simulink model "walk2"  (R2020a)
settings: Solver=FixedStepDiscrete  StartTime=0.0  StopTime=20  FixedStep=deltaT  RelTol=1e-3
InitFcn:
  | %****NOTE: you must change the line below
  | % to the IP address for YOUR ROS master!****
  | deltaT = 0.1;
  | %ipaddress = 'http://10.4.155.40:11311'; % Tech Hall
  | ipaddress = 'http://192.168.43.20:11311'; % phone
  | 
  | % --- Start MATLAB Global Node
  | try % try to print list of ROS nodes
  |     rosnode list
  |     clc
  | % if error from rosnode list,
  | % initialize ROS global node from MATLAB
  | catch exp
  |     rosinit(ipaddress)  % only if error: rosinit
  |     pause(5)
  | end
StartFcn:
  | % Publishers to ROS topics for left, right
  | % upper arm joint commands
  | Larm = rospublisher('/darwin/j_high_arm_l_position_controller/command','std_msgs/Float64');
  | Rarm = rospublisher('/darwin/j_high_arm_r_position_controller/command','std_msgs/Float64');
  | 
  | % Create ROS messages to publishers
  | Ldown = rosmessage(Larm);
  | Rdown = rosmessage(Rarm);
  | Ldown2 = rosmessage(Larm);
  | Rdown2 = rosmessage(Rarm);
  | 
  | % move upper arm joint to 0.5 radian
  | Ldown.Data = 0.5;
  | Rdown.Data = 0.5;
  | 
  | % move upper arm joint to 0.8 radian
  | Ldown2.Data = 0.8;
  | Rdown2.Data = 0.8;
  | 
  | % move arms to 0.5 radian during two-second period,
  | % then to 0.8 radian during another
  | % two-second period (arms move synchronously)
  | send(Larm,Ldown);
  | send(Rarm,Rdown);
  | pause(2)
  | send(Larm,Ldown2);
  | send(Rarm,Rdown2);
  | pause(2)
  | 
  | disturb = rossvcclient('/gazebo/apply_body_wrench');
  | disturbmsg = rosmessage(disturb);
  | disturbmsg.ReferenceFrame = 'world';
  | disturbmsg.ReferencePoint.X = 0; disturbmsg.ReferencePoint.Y = 0; disturbmsg.ReferencePoint.Z = 0;
  | disturbmsg.Wrench.Force.X = 0.0; disturbmsg.Wrench.Force.Y = 0.0; disturbmsg.Wrench.Force.Z = 0.0;
  | disturbmsg.Wrench.Torque.X = 0.0; disturbmsg.Wrench.Torque.Y = 0.0; disturbmsg.Wrench.Torque.Z = 0.0;
  | disturbmsg.StartTime.Sec = 0; disturbmsg.StartTime.Nsec = 0;
  | disturbmsg.Duration.Sec = 0; disturbmsg.Duration.Nsec = 500000000;
StopFcn:
  | rosshutdown
model workspace (MAT data in the model file):
  SL_ROS_VariableLengthArrays_MaxSizes.CommonInfo.ArrayTruncateAction = 'EmitWarning'
  SL_ROS_VariableLengthArrays_MaxSizes.MsgTypeMap = containers.Map
  SL_ROS_VariableLengthArrays_MaxSizes.MsgTypeMap.serialization.keys = {'gazebo_msgs/ApplyBodyWrenchRequest', 'sensor_msgs/JointState'}
  SL_ROS_VariableLengthArrays_MaxSizes.MsgTypeMap.serialization.values{1}(1).PropertyName = 'BodyName'
  SL_ROS_VariableLengthArrays_MaxSizes.MsgTypeMap.serialization.values{1}(1).DataType = 'uint8'
  SL_ROS_VariableLengthArrays_MaxSizes.MsgTypeMap.serialization.values{1}(1).MaxLength = 19
  SL_ROS_VariableLengthArrays_MaxSizes.MsgTypeMap.serialization.values{1}(2).PropertyName = 'ReferenceFrame'
  SL_ROS_VariableLengthArrays_MaxSizes.MsgTypeMap.serialization.values{1}(2).DataType = 'uint8'
  SL_ROS_VariableLengthArrays_MaxSizes.MsgTypeMap.serialization.values{1}(2).MaxLength = 5
  SL_ROS_VariableLengthArrays_MaxSizes.MsgTypeMap.serialization.values{2}(1).PropertyName = 'Effort'
  SL_ROS_VariableLengthArrays_MaxSizes.MsgTypeMap.serialization.values{2}(1).DataType = 'double'
  SL_ROS_VariableLengthArrays_MaxSizes.MsgTypeMap.serialization.values{2}(1).MaxLength = 128
  SL_ROS_VariableLengthArrays_MaxSizes.MsgTypeMap.serialization.values{2}(2).PropertyName = 'Name'
  SL_ROS_VariableLengthArrays_MaxSizes.MsgTypeMap.serialization.values{2}(2).DataType = 'std_msgs/String'
  SL_ROS_VariableLengthArrays_MaxSizes.MsgTypeMap.serialization.values{2}(2).MaxLength = 24
  SL_ROS_VariableLengthArrays_MaxSizes.MsgTypeMap.serialization.values{2}(3).PropertyName = 'Position'
  SL_ROS_VariableLengthArrays_MaxSizes.MsgTypeMap.serialization.values{2}(3).DataType = 'double'
  SL_ROS_VariableLengthArrays_MaxSizes.MsgTypeMap.serialization.values{2}(3).MaxLength = 128
  SL_ROS_VariableLengthArrays_MaxSizes.MsgTypeMap.serialization.values{2}(4).PropertyName = 'Velocity'
  SL_ROS_VariableLengthArrays_MaxSizes.MsgTypeMap.serialization.values{2}(4).DataType = 'double'
  SL_ROS_VariableLengthArrays_MaxSizes.MsgTypeMap.serialization.values{2}(4).MaxLength = 128
  SL_ROS_VariableLengthArrays_MaxSizes.MsgTypeMap.serialization.uniformity = 0
  SL_ROS_VariableLengthArrays_MaxSizes.MsgTypeMap.serialization.keyType = 'char'
  SL_ROS_VariableLengthArrays_MaxSizes.MsgTypeMap.serialization.valueType = 'any'
libraries: robotlib x22, realtime_pacer_lib x1
settings Model: Creator=JerryLee  LastModifiedBy=JerryLee
settings OptimizationCC: EnhancedBackFolding=on  PassReuseOutputArgsAs=Individual arguments  ZeroExternalMemoryAtStartup=off  ZeroInternalMemoryAtStartup=off  MaxStackSize=64  OptimizeBlockOrder=speed  DifferentSizesBufferReuse=on  OptimizationCustomize=off  EfficientTunableParamExpr=on
settings DebuggingCC: ParameterTunabilityLossMsg=error
settings HardwareCC: ProdBitPerPointer=32  ProdBitPerSizeT=32  ProdBitPerPtrDiffT=32  ProdLargestAtomicFloat=None  ProdIntDivRoundTo=Undefined  ProdEndianess=Unspecified  ProdWordSize=32  ProdHWDeviceType=Generic->Unspecified (assume 32-bit Generic)  UseEmbeddedCoderFeatures=off
settings SFSimCC: MATLABDynamicMemAlloc=off
settings RTWCC: SystemTargetFile=ert.tlc  HardwareBoard=Robot Operating System (ROS)  TemplateMakefile=ert_default_tmf  Toolchain=Catkin  TargetLang=C++
settings CodeAppCC: ForceParamTrailComments=on  IgnoreCustomStorageClasses=off  OperatorAnnotations=on  SimulinkDataObjDesc=on  SFDataObjDesc=on  InsertBlockDesc=on
settings ERTTargetCC: SupportNonInlinedSFcns=on

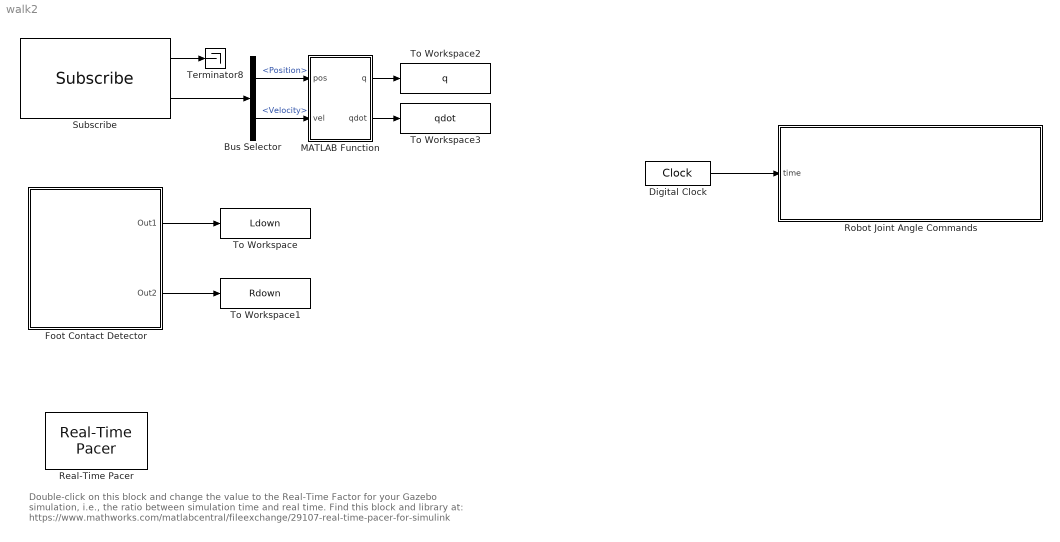
== system walk2 ==
  note: Double-click on this block and
      | change the value to the Real-Time
      | Factor for your Gazebo simulation,
      | i.e., the ratio between simulation time
      | and real time.
      |
      | Find this block and library at:
      | https://www.mathworks.com/matlabcentral/fileexchange/29107-real-time-pacer-for-simulink
  Bus Selector : BusSelector  OutputSignals=Position,Velocity
  Digital Clock : DigitalClock  SampleTime=deltaT
  Foot Contact Detector : Subsystem
  MATLAB Function : MATLAB Function  TreatAsAtomicUnit=on
  Real-Time Pacer : realtime_pacer_lib/Real-Time Pacer  simTimePerRealTime=0.5
      settings: SourceProductName=Real-Time Pacer
  Robot Joint Angle Commands : Subsystem
  Subscribe : robotlib/Subscribe  topicSource=Select from ROS network  topic=/darwin/joint_states  messageType=sensor_msgs/JointState  sampleTime=deltaT  messageQueueLength=1
  Terminator8 : Terminator
  To Workspace : ToWorkspace  VariableName=Ldown  SampleTime=deltaT
  To Workspace1 : ToWorkspace  VariableName=Rdown  SampleTime=deltaT
  To Workspace2 : ToWorkspace  VariableName=q  SampleTime=deltaT
  To Workspace3 : ToWorkspace  VariableName=qdot  SampleTime=deltaT
  wires:
  Subscribe/1 -> Terminator8/1
  Foot Contact Detector/2(Out2) -> To Workspace1/1
  Foot Contact Detector/1(Out1) -> To Workspace/1
  Subscribe/2 -> Bus Selector/1
  Digital Clock/1 -> Robot Joint Angle Commands/1(time)
  Bus Selector/1 -> MATLAB Function/1(pos)  "<Position>"
  Bus Selector/2 -> MATLAB Function/2(vel)  "<Velocity>"
  MATLAB Function/1(q) -> To Workspace2/1
  MATLAB Function/2(qdot) -> To Workspace3/1

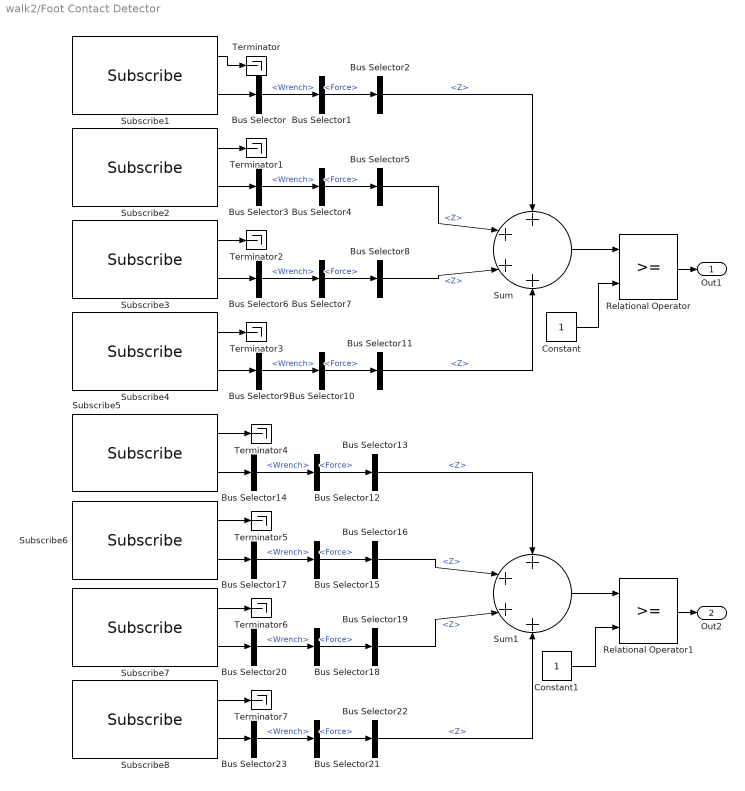
== system walk2/Foot Contact Detector ==
  Bus Selector{,3,6,9,14,17,20,23} (8 alike) : BusSelector  OutputSignals=Wrench
  Bus Selector{1,4,7,10,12,15,18,21} (8 alike) : BusSelector  OutputSignals=Force
  Bus Selector{2,5,8,11,13,16,19,22} (8 alike) : BusSelector  OutputSignals=Z
  Constant : Constant
  Constant1 : Constant
  Relational Operator : RelationalOperator  OutDataTypeStr=boolean  RndMeth=Simplest
  Relational Operator1 : RelationalOperator  OutDataTypeStr=boolean  RndMeth=Simplest
  Subscribe1 : robotlib/Subscribe  topicSource=Select from ROS network  topic=/leap_one/left_foot_sensor_m0  messageType=geometry_msgs/WrenchStamped  sampleTime=deltaT  messageQueueLength=1
  Subscribe2 : robotlib/Subscribe  topicSource=Select from ROS network  topic=/leap_one/left_foot_sensor_m1  messageType=geometry_msgs/WrenchStamped  sampleTime=deltaT  messageQueueLength=1
  Subscribe3 : robotlib/Subscribe  topicSource=Select from ROS network  topic=/leap_one/left_foot_sensor_m2  messageType=geometry_msgs/WrenchStamped  sampleTime=deltaT  messageQueueLength=1
  Subscribe4 : robotlib/Subscribe  topicSource=Select from ROS network  topic=/leap_one/left_foot_sensor_m3  messageType=geometry_msgs/WrenchStamped  sampleTime=deltaT  messageQueueLength=1
  Subscribe5 : robotlib/Subscribe  topicSource=Select from ROS network  topic=/leap_one/right_foot_sensor_m0  messageType=geometry_msgs/WrenchStamped  sampleTime=deltaT  messageQueueLength=1
  Subscribe6 : robotlib/Subscribe  topicSource=Select from ROS network  topic=/leap_one/right_foot_sensor_m1  messageType=geometry_msgs/WrenchStamped  sampleTime=deltaT  messageQueueLength=1
  Subscribe7 : robotlib/Subscribe  topicSource=Select from ROS network  topic=/leap_one/right_foot_sensor_m2  messageType=geometry_msgs/WrenchStamped  sampleTime=deltaT  messageQueueLength=1
  Subscribe8 : robotlib/Subscribe  topicSource=Select from ROS network  topic=/leap_one/right_foot_sensor_m3  messageType=geometry_msgs/WrenchStamped  sampleTime=deltaT  messageQueueLength=1
  Sum : Sum  Inputs=4
  Sum1 : Sum  Inputs=4
  Terminator{,1..7} (8 alike) : Terminator
  Out1 : Outport
  Out2 : Outport  Port=2
  wires:
  Bus Selector6/1 -> Bus Selector7/1  "<Wrench>"
  Subscribe8/2 -> Bus Selector23/1
  Bus Selector22/1 -> Sum1/4  "<Z>"
  Bus Selector8/1 -> Sum/3  "<Z>"
  Subscribe5/1 -> Terminator4/1
  Bus Selector/1 -> Bus Selector1/1  "<Wrench>"
  Subscribe1/2 -> Bus Selector/1
  Bus Selector2/1 -> Sum/1  "<Z>"
  Bus Selector20/1 -> Bus Selector18/1  "<Wrench>"
  Bus Selector19/1 -> Sum1/3  "<Z>"
  Subscribe2/2 -> Bus Selector3/1
  Bus Selector17/1 -> Bus Selector15/1  "<Wrench>"
  Constant/1 -> Relational Operator/2
  Bus Selector3/1 -> Bus Selector4/1  "<Wrench>"
  Relational Operator1/1 -> Out2/1
  Bus Selector18/1 -> Bus Selector19/1  "<Force>"
  Bus Selector9/1 -> Bus Selector10/1  "<Wrench>"
  Subscribe2/1 -> Terminator1/1
  Bus Selector4/1 -> Bus Selector5/1  "<Force>"
  Bus Selector16/1 -> Sum1/2  "<Z>"
  Subscribe7/1 -> Terminator6/1
  Relational Operator/1 -> Out1/1
  Bus Selector13/1 -> Sum1/1  "<Z>"
  Constant1/1 -> Relational Operator1/2
  Subscribe7/2 -> Bus Selector20/1
  Bus Selector23/1 -> Bus Selector21/1  "<Wrench>"
  Subscribe6/2 -> Bus Selector17/1
  Subscribe6/1 -> Terminator5/1
  Bus Selector10/1 -> Bus Selector11/1  "<Force>"
  Bus Selector21/1 -> Bus Selector22/1  "<Force>"
  Sum/1 -> Relational Operator/1
  Subscribe3/1 -> Terminator2/1
  Bus Selector11/1 -> Sum/4  "<Z>"
  Bus Selector5/1 -> Sum/2  "<Z>"
  Subscribe4/2 -> Bus Selector9/1
  Subscribe5/2 -> Bus Selector14/1
  Subscribe3/2 -> Bus Selector6/1
  Bus Selector7/1 -> Bus Selector8/1  "<Force>"
  Subscribe1/1 -> Terminator/1
  Sum1/1 -> Relational Operator1/1
  Bus Selector15/1 -> Bus Selector16/1  "<Force>"
  Bus Selector1/1 -> Bus Selector2/1  "<Force>"
  Subscribe4/1 -> Terminator3/1
  Bus Selector14/1 -> Bus Selector12/1  "<Wrench>"
  Subscribe8/1 -> Terminator7/1
  Bus Selector12/1 -> Bus Selector13/1  "<Force>"

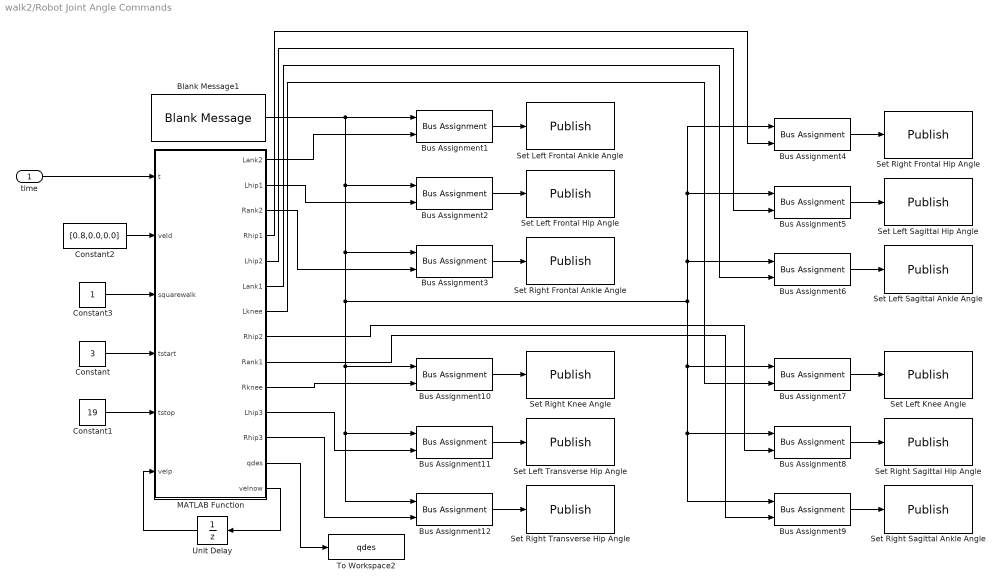
== system walk2/Robot Joint Angle Commands ==
  time : Inport
  Blank Message1 : robotlib/Blank Message  messageClass=Message  entityType=std_msgs/Float64  messageType=std_msgs/Float64  SampleTime=deltaT
  Bus Assignment{1..12} (12 alike) : BusAssignment  AssignedSignals=Data
  Constant : Constant  Value=3
  Constant1 : Constant  Value=19
  Constant2 : Constant  Value=[0.8,0.0,0.0]
  Constant3 : Constant
  MATLAB Function : MATLAB Function  TreatAsAtomicUnit=on
  Set Left Frontal Ankle Angle : robotlib/Publish  topicSource=Select from ROS network  topic=/darwin/j_ankle2_l_position_controller/command  messageType=std_msgs/Float64  messageQueueLength=1
  Set Left Frontal Hip Angle : robotlib/Publish  topicSource=Select from ROS network  topic=/darwin/j_thigh1_l_position_controller/command  messageType=std_msgs/Float64  messageQueueLength=1
  Set Left Knee Angle : robotlib/Publish  topicSource=Select from ROS network  topic=/darwin/j_tibia_l_position_controller/command  messageType=std_msgs/Float64  messageQueueLength=1
  Set Left Sagittal Ankle Angle : robotlib/Publish  topicSource=Select from ROS network  topic=/darwin/j_ankle1_l_position_controller/command  messageType=std_msgs/Float64  messageQueueLength=1
  Set Left Sagittal Hip Angle : robotlib/Publish  topicSource=Select from ROS network  topic=/darwin/j_thigh2_l_position_controller/command  messageType=std_msgs/Float64  messageQueueLength=1
  Set Left Transverse Hip Angle : robotlib/Publish  topicSource=Select from ROS network  topic=/darwin/j_pelvis_l_position_controller/command  messageType=std_msgs/Float64  messageQueueLength=1
  Set Right Frontal Ankle Angle : robotlib/Publish  topicSource=Select from ROS network  topic=/darwin/j_ankle2_r_position_controller/command  messageType=std_msgs/Float64  messageQueueLength=1
  Set Right Frontal Hip Angle : robotlib/Publish  topicSource=Select from ROS network  topic=/darwin/j_thigh1_r_position_controller/command  messageType=std_msgs/Float64  messageQueueLength=1
  Set Right Knee Angle : robotlib/Publish  topicSource=Select from ROS network  topic=/darwin/j_tibia_r_position_controller/command  messageType=std_msgs/Float64  messageQueueLength=1
  Set Right Sagittal Ankle Angle : robotlib/Publish  topicSource=Select from ROS network  topic=/darwin/j_ankle1_r_position_controller/command  messageType=std_msgs/Float64  messageQueueLength=1
  Set Right Sagittal Hip Angle : robotlib/Publish  topicSource=Select from ROS network  topic=/darwin/j_thigh2_r_position_controller/command  messageType=std_msgs/Float64  messageQueueLength=1
  Set Right Transverse Hip Angle : robotlib/Publish  topicSource=Select from ROS network  topic=/darwin/j_pelvis_r_position_controller/command  messageType=std_msgs/Float64  messageQueueLength=1
  To Workspace2 : ToWorkspace  VariableName=qdes  SampleTime=deltaT
  Unit Delay : UnitDelay  InitialCondition=[0,0,0]  SampleTime=-1  HasFrameUpgradeWarning=on
  wires:
  Bus Assignment1/1 -> Set Left Frontal Ankle Angle/1
  Bus Assignment2/1 -> Set Left Frontal Hip Angle/1
  Bus Assignment3/1 -> Set Right Frontal Ankle Angle/1
  Bus Assignment6/1 -> Set Left Sagittal Ankle Angle/1
  Bus Assignment5/1 -> Set Left Sagittal Hip Angle/1
  Bus Assignment4/1 -> Set Right Frontal Hip Angle/1
  Bus Assignment10/1 -> Set Right Knee Angle/1
  Bus Assignment11/1 -> Set Left Transverse Hip Angle/1
  Bus Assignment12/1 -> Set Right Transverse Hip Angle/1
  Bus Assignment9/1 -> Set Right Sagittal Ankle Angle/1
  Bus Assignment8/1 -> Set Right Sagittal Hip Angle/1
  Bus Assignment7/1 -> Set Left Knee Angle/1
  Blank Message1/1 -> Bus Assignment11/1, Bus Assignment12/1, Bus Assignment10/1, Bus Assignment9/1, Bus Assignment8/1, Bus Assignment7/1, Bus Assignment6/1, Bus Assignment5/1, Bus Assignment4/1, Bus Assignment3/1, Bus Assignment2/1, Bus Assignment1/1
  time/1 -> MATLAB Function/1(t)
  MATLAB Function/14(velnow) -> Unit Delay/1
  Unit Delay/1 -> MATLAB Function/6(velp)
  MATLAB Function/1(Lank2) -> Bus Assignment1/2
  MATLAB Function/2(Lhip1) -> Bus Assignment2/2
  MATLAB Function/3(Rank2) -> Bus Assignment3/2
  MATLAB Function/12(Rhip3) -> Bus Assignment12/2
  MATLAB Function/11(Lhip3) -> Bus Assignment11/2
  MATLAB Function/10(Rknee) -> Bus Assignment10/2
  MATLAB Function/9(Rank1) -> Bus Assignment9/2
  MATLAB Function/8(Rhip2) -> Bus Assignment8/2
  MATLAB Function/7(Lknee) -> Bus Assignment7/2
  MATLAB Function/6(Lank1) -> Bus Assignment6/2
  MATLAB Function/5(Lhip2) -> Bus Assignment5/2
  MATLAB Function/4(Rhip1) -> Bus Assignment4/2
  Constant/1 -> MATLAB Function/4(tstart)
  Constant1/1 -> MATLAB Function/5(tstop)
  Constant2/1 -> MATLAB Function/2(veld)
  MATLAB Function/13(qdes) -> To Workspace2/1
  Constant3/1 -> MATLAB Function/3(squarewalk)

== matlab function walk2/Robot Joint Angle Commands/MATLAB Function ==
  data: Lank2 output; t input; veld input; squarewalk input; tstart input; tstop input; Lhip1 output; Rank2 output; Rhip1 output; Lhip2 output; Lank1 output; Lknee output; Rhip2 output; Rank1 output; Rknee output; Lhip3 output; Rhip3 output; qdes output; velnow output; velp input
function [Lank2,Lhip1,Rank2,Rhip1,Lhip2,Lank1,Lknee,Rhip2,Rank1,Rknee,Lhip3,Rhip3,qdes,velnow] = fcn(t,veld,squarewalk,tstart,tstop,velp)
% inputs: current time 't', desired gait velocity vector 'veldes': [x vel,y vel,z ang vel]
% gait start time 'tstart', gait command stop time 'tstop', previous gait velocity 'velp'
% outputs: desired joint angles for 12 DOF of lower body of DARwIn, most current
% estimate of joint velocity 'velnow'
veldes = [veld(1),veld(2),veld(3)];
velprev = [velp(1),velp(2),velp(3)];
dt = 0.1;
n = 5;

if squarewalk ~= 1
    if t < tstart || (t >= tstop && norm(velprev) < 0.1)
        phase = 1; % 'phase' = 1 represents second half of cycle before the one commencing at 'tstart'
        velnow = [0.0,0.0,0.0]; % current velocity should be zero before 'tstart'
        x = 0; % since cycle has not started yet, the ratio of phase that is completed is zero
    else
        c = floor((t-tstart)/dt); % number of "timesteps" of duration dt since 'tstart'
        
        % determine whether, according to time, the robot is in the first ('phase' = 0) or
        % second ('phase' = 1) half of the gait cycle:
        if mod(floor(c/n),2) == 1
            phase = 0;
        else
            phase = 1;
        end
        x = mod(c,n)/n; % ratio of phase completed 

        % if time has elapsed past 'tstop'...
        if t >= tstop
            veldes = [0.0,0.0,0.0]; % set desired velocity equal to zero
        end

        % update current estimate of gait velocity
        velnow = (3/n)*veldes + (1 - (3/n))*velprev;
    end
else % if robot is walking in predetermined square pattern...
    if t < tstart || (t >= tstop && norm(velprev) < 0.1)
        phase = 1; % 'phase' = 1 represents second half of cycle before the one commencing at 'tstart'
        velnow = [0.0,0.0,0.0]; % current velocity should be zero before 'tstart'
        x = 0; % since cycle has not started yet, the ratio of phase that is completed is zero
    else
        if t < 0.75*tstart + 0.25*tstop
            c = floor((t-tstart)/dt); % number of "timesteps" of duration dt since 'tstart'
            veldes = [0.0,0.4,0.0]; % walk left for first 1/4 of walk time
            % determine whether, according to time, the robot is in the first ('phase' = 0) or
            % second ('phase' = 1) half of the gait cycle:
            if mod(floor(c/n),2) == 1
                phase = 0;
            else
                phase = 1;
            end
            x = mod(c,n)/n; % ratio of phase completed 

            % update current estimate of gait velocity
            velnow = (3/n)*veldes + (1 - (3/n))*velprev;

        else
            if t < 0.5*tstart + 0.5*tstop
                c = floor((t-(0.75*tstart + 0.25*tstop))/dt); % number of "timesteps" of duration dt since 'tstart'
                veldes = [-0.4,0.0,0.0]; % walk backward for second 1/4 of walk time
                % determine whether, according to time, the robot is in the first ('phase' = 0) or
                % second ('phase' = 1) half of the gait cycle:
                if mod(floor(c/n),2) == 1
                    phase = 0;
                else
                    phase = 1;
                end
                x = mod(c,n)/n; % ratio of phase completed 

                % update current estimate of gait velocity
                velnow = (3/n)*veldes + (1 - (3/n))*velprev;

            else
                if t < 0.25*tstart + 0.75*tstop
                    c = floor((t-(0.5*tstart + 0.5*tstop))/dt); % number of "timesteps" of duration dt since 'tstart'
                    veldes = [0.0,-0.4,0.0]; % walk right for third 1/4 of walk time
                    % determine whether, according to time, the robot is in the first ('phase' = 0) or
                    % second ('phase' = 1) half of the gait cycle:
                    if mod(floor(c/n),2) == 1
                        phase = 0;
                    else
                        phase = 1;
                    end
                    x = mod(c,n)/n; % ratio of phase completed 

                    % update current estimate of gait velocity
                    velnow = (3/n)*veldes + (1 - (3/n))*velprev;
                else
                    c = floor((t-(0.25*tstart + 0.75*tstop))/dt); % number of "timesteps" of duration dt since 'tstart'
                    veldes = [0.4,0.0,0.0]; % walk forward for final 1/4 of walk time
                    % determine whether, according to time, the robot is in the first ('phase' = 0) or
                    % second ('phase' = 1) half of the gait cycle:
                    if mod(floor(c/n),2) == 1
                        phase = 0;
                    else
                        phase = 1;
                    end
                    x = mod(c,n)/n; % ratio of phase completed 

                    % if time has elapsed past 'tstop'...
                    if t >= tstop
                        veldes = [0.0,0.0,0.0]; % set desired velocity equal to zero
                    end

                    % update current estimate of gait velocity
                    velnow = (3/n)*veldes + (1 - (3/n))*velprev;   
                end
            end
        end
    end
    
end

[p,a,params] = MultiCPG([]); % generate phase and antiphase gait functions
angles = [GetJointAngles(p,a,params,phase,x,velnow);phase]; % compute desired joint angles

% assign computed joint angle vector values to appropriate variables
Lank2 = angles(1); Lhip1 = angles(2); Rank2 = angles(3);
Rhip1 = angles(4); Lhip2 = angles(5); Lank1 = angles(6);
Lknee = angles(7); Rhip2 = angles(8); Rank1 = angles(9);
Rknee = angles(10); Lhip3 = angles(11); Rhip3 = angles(12);

qdes = angles(1:12);

== matlab function walk2/MATLAB Function ==
  data: q output; pos input; vel input; qdot output
function [q,qdot] = fcn(pos,vel)
% inputs: current position and velocity outputs from ROS message
% outputs: truncated, rearranged position, velocity vectors

% position/velocity vectors have values for joints in this order:
% Lankle1, Rankle1, Lankle2, Rankle2, Lgripper*, Rgripper*
% Lshoulder2*, Rshoulder2*, Lelbow*, Relbow*, Neck*, Lhip3, Rhip3,
% Lshoulder1*, Rshoulder1*, Lhip1, Rhip1, Lhip2, Rhip2, Lknee, Rknee, 
% Camera*, Lwrist*, Rwrist*
% (for lower-body control, we only use 12 of these 24, not the starred ones)

q = zeros(12,1);
qdot = zeros(12,1);

q(1) = pos(3); q(2) = pos(16); q(3) = pos(4); q(4) = pos(17);
q(5) = pos(18); q(6) = pos(1); q(7) = pos(20); q(8) = pos(19);
q(9) = pos(2); q(10) = pos(21); q(11) = pos(12); q(12) = pos(13);

qdot(1) = vel(3); qdot(2) = vel(16); qdot(3) = vel(4); qdot(4) = vel(17);
qdot(5) = vel(18); qdot(6) = vel(1); qdot(7) = vel(20); qdot(8) = vel(19);
qdot(9) = vel(2); qdot(10) = vel(21); qdot(11) = vel(12); qdot(12) = vel(13);
